simulink model "MAIN_SAT_PID"  (R2018b)
settings: Solver=FixedStepAuto  StartTime=0.0  StopTime=10.0  FixedStep=0.01  RelTol=1e-3
libraries: simulink x3
settings Model: Creator=22672  LastModifiedBy=cx

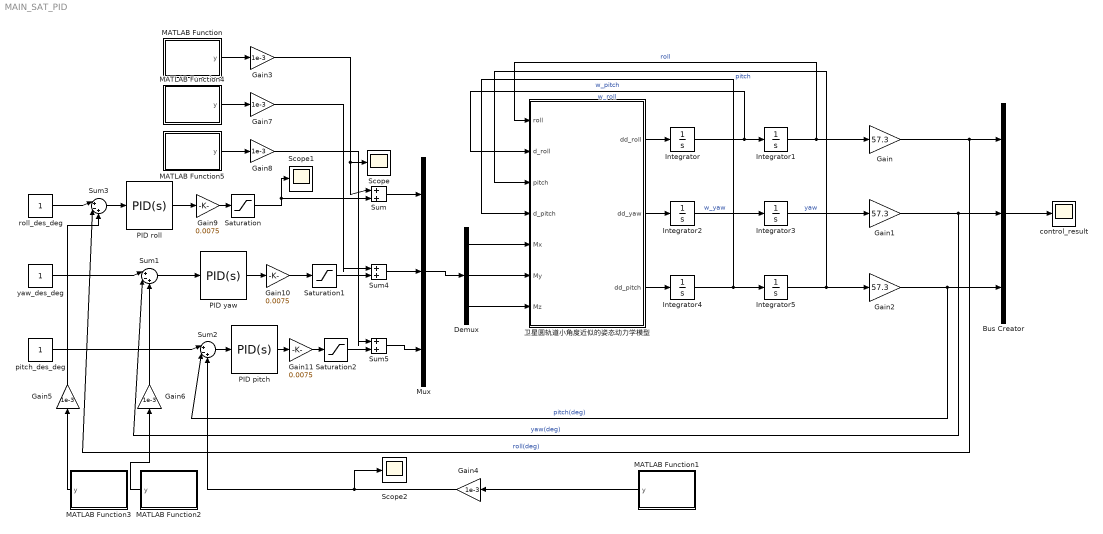
== system MAIN_SAT_PID ==
  Bus Creator : BusCreator  Inputs=3
  Demux : Demux  Outputs=3
  Gain : Gain  Gain=57.3
  Gain1 : Gain  Gain=57.3
  Gain10 : Gain  Gain=0.0075
  Gain11 : Gain  Gain=0.0075
  Gain2 : Gain  Gain=57.3
  Gain{3..8} (6 alike) : Gain  Gain=1e-3
  Gain9 : Gain  Gain=0.0075
  Integrator{,1..5} (6 alike) : Integrator
  MATLAB Function : MATLAB Function  TreatAsAtomicUnit=on
  MATLAB Function1 : MATLAB Function  TreatAsAtomicUnit=on
  MATLAB Function2 : MATLAB Function  TreatAsAtomicUnit=on
  MATLAB Function3 : MATLAB Function  TreatAsAtomicUnit=on
  MATLAB Function4 : MATLAB Function  TreatAsAtomicUnit=on
  MATLAB Function5 : MATLAB Function  TreatAsAtomicUnit=on
  Mux : Mux  Inputs=3
  PID pitch : simulink/Continuous/PID Controller  Controller=PID  Form=Parallel  TimeDomain=Continuous-time  SampleTime=-1  IntegratorMethod=Forward Euler  FilterMethod=Forward Euler  ControllerParametersSource=internal  P=22  I=0  D=14.2  UseFilter=on  N=100  TunerSelectOption=Transfer Function Based (PID Tuner App)  InitialConditionSource=internal  InitialConditionForIntegrator=0  InitialConditionForFilter=0  DifferentiatorICPrevScaledInput=0  ExternalReset=none  TrackingMode=off  Kt=1  LimitOutput=off  UpperSaturationLimit=inf  LowerSaturationLimit=-inf  LinearizeAsGain=on  AntiWindupMode=none  Kb=1  POutMin=[]  POutMax=[]  IOutMin=[]  IOutMax=[]  DOutMin=[]  DOutMax=[]  NOutMin=[]  NOutMax=[]  SumOutMin=[]  SumOutMax=[]  SaturationOutMin=[]  SaturationOutMax=[]  PParamMin=[]  PParamMax=[]  IParamMin=[]  IParamMax=[]  DParamMin=[]  DParamMax=[]  NParamMin=[]  NParamMax=[]  KbParamMin=[]  KbParamMax=[]  KtParamMin=[]  KtParamMax=[]  KbOutMin=[]  KbOutMax=[]  KtOutMin=[]  KtOutMax=[]  IntegratorOutMin=[]  IntegratorOutMax=[]  FilterOutMin=[]  FilterOutMax=[]  SumI1OutMin=[]  SumI1OutMax=[]  SumI2OutMin=[]  SumI2OutMax=[]  SumI3OutMin=[]  SumI3OutMax=[]  SumI4OutMin=[]  SumI4OutMax=[]  SumDOutMin=[]  SumDOutMax=[]  DifferentiatorOutMin=[]  DifferentiatorOutMax=[]  FilterDiffOutCoefMin=[]  FilterDiffOutCoefMax=[]  ReciprocalOutMin=[]  ReciprocalOutMax=[]  SumDenOutMin=[]  SumDenOutMax=[]  SumNumOutMin=[]  SumNumOutMax=[]  DivideOutMin=[]  DivideOutMax=[]  IntegratorContinuousStateAttributes=''  IntegratorStateMustResolveToSignalObject=off  IntegratorRTWStateStorageClass=Auto  FilterContinuousStateAttributes=''  FilterStateMustResolveToSignalObject=off  FilterRTWStateStorageClass=Auto  ParallelPVariant=InternalParameters  IdealPVariant=Disabled  IVariant=InternalParameters  DVariant=InternalParameters  IntegratorVariant=Continuous  SatVariant=Disabled  AWVariant=Passthrough  PCopyVariant=Disabled  TRVariant=Disabled  FdbkBlocksVariant=Forward  IdealPFdbkVariant=Disabled  SatFdbkVariant=Disabled  DerivativeFilterVariant=ContFilter  NVariant=InternalParameters  NCopyVariant=Disabled  FilterICVariant=InternalICsFilter  IntegratorICVariant=InternalICs  ExternalResetVariant=Disabled  TRSumVariant=Passthrough  SumFdbkVariant=Disabled  SumVariant=Sum_PID
  PID roll : simulink/Continuous/PID Controller  Controller=PID  Form=Parallel  TimeDomain=Continuous-time  SampleTime=-1  IntegratorMethod=Forward Euler  FilterMethod=Forward Euler  ControllerParametersSource=internal  P=40  I=0  D=12  UseFilter=on  N=100  TunerSelectOption=Transfer Function Based (PID Tuner App)  InitialConditionSource=internal  InitialConditionForIntegrator=0  InitialConditionForFilter=0  DifferentiatorICPrevScaledInput=0  ExternalReset=none  TrackingMode=off  Kt=1  LimitOutput=off  UpperSaturationLimit=inf  LowerSaturationLimit=-inf  LinearizeAsGain=on  AntiWindupMode=none  Kb=1  POutMin=[]  POutMax=[]  IOutMin=[]  IOutMax=[]  DOutMin=[]  DOutMax=[]  NOutMin=[]  NOutMax=[]  SumOutMin=[]  SumOutMax=[]  SaturationOutMin=[]  SaturationOutMax=[]  PParamMin=[]  PParamMax=[]  IParamMin=[]  IParamMax=[]  DParamMin=[]  DParamMax=[]  NParamMin=[]  NParamMax=[]  KbParamMin=[]  KbParamMax=[]  KtParamMin=[]  KtParamMax=[]  KbOutMin=[]  KbOutMax=[]  KtOutMin=[]  KtOutMax=[]  IntegratorOutMin=[]  IntegratorOutMax=[]  FilterOutMin=[]  FilterOutMax=[]  SumI1OutMin=[]  SumI1OutMax=[]  SumI2OutMin=[]  SumI2OutMax=[]  SumI3OutMin=[]  SumI3OutMax=[]  SumI4OutMin=[]  SumI4OutMax=[]  SumDOutMin=[]  SumDOutMax=[]  DifferentiatorOutMin=[]  DifferentiatorOutMax=[]  FilterDiffOutCoefMin=[]  FilterDiffOutCoefMax=[]  ReciprocalOutMin=[]  ReciprocalOutMax=[]  SumDenOutMin=[]  SumDenOutMax=[]  SumNumOutMin=[]  SumNumOutMax=[]  DivideOutMin=[]  DivideOutMax=[]  IntegratorContinuousStateAttributes=''  IntegratorStateMustResolveToSignalObject=off  IntegratorRTWStateStorageClass=Auto  FilterContinuousStateAttributes=''  FilterStateMustResolveToSignalObject=off  FilterRTWStateStorageClass=Auto  ParallelPVariant=InternalParameters  IdealPVariant=Disabled  IVariant=InternalParameters  DVariant=InternalParameters  IntegratorVariant=Continuous  SatVariant=Disabled  AWVariant=Passthrough  PCopyVariant=Disabled  TRVariant=Disabled  FdbkBlocksVariant=Forward  IdealPFdbkVariant=Disabled  SatFdbkVariant=Disabled  DerivativeFilterVariant=ContFilter  NVariant=InternalParameters  NCopyVariant=Disabled  FilterICVariant=InternalICsFilter  IntegratorICVariant=InternalICs  ExternalResetVariant=Disabled  TRSumVariant=Passthrough  SumFdbkVariant=Disabled  SumVariant=Sum_PID
  PID yaw : simulink/Continuous/PID Controller  Controller=PID  Form=Parallel  TimeDomain=Continuous-time  SampleTime=-1  IntegratorMethod=Forward Euler  FilterMethod=Forward Euler  ControllerParametersSource=internal  P=30  I=0  D=13.67  UseFilter=on  N=100  TunerSelectOption=Transfer Function Based (PID Tuner App)  InitialConditionSource=internal  InitialConditionForIntegrator=0  InitialConditionForFilter=0  DifferentiatorICPrevScaledInput=0  ExternalReset=none  TrackingMode=off  Kt=1  LimitOutput=off  UpperSaturationLimit=inf  LowerSaturationLimit=-inf  LinearizeAsGain=on  AntiWindupMode=none  Kb=1  POutMin=[]  POutMax=[]  IOutMin=[]  IOutMax=[]  DOutMin=[]  DOutMax=[]  NOutMin=[]  NOutMax=[]  SumOutMin=[]  SumOutMax=[]  SaturationOutMin=[]  SaturationOutMax=[]  PParamMin=[]  PParamMax=[]  IParamMin=[]  IParamMax=[]  DParamMin=[]  DParamMax=[]  NParamMin=[]  NParamMax=[]  KbParamMin=[]  KbParamMax=[]  KtParamMin=[]  KtParamMax=[]  KbOutMin=[]  KbOutMax=[]  KtOutMin=[]  KtOutMax=[]  IntegratorOutMin=[]  IntegratorOutMax=[]  FilterOutMin=[]  FilterOutMax=[]  SumI1OutMin=[]  SumI1OutMax=[]  SumI2OutMin=[]  SumI2OutMax=[]  SumI3OutMin=[]  SumI3OutMax=[]  SumI4OutMin=[]  SumI4OutMax=[]  SumDOutMin=[]  SumDOutMax=[]  DifferentiatorOutMin=[]  DifferentiatorOutMax=[]  FilterDiffOutCoefMin=[]  FilterDiffOutCoefMax=[]  ReciprocalOutMin=[]  ReciprocalOutMax=[]  SumDenOutMin=[]  SumDenOutMax=[]  SumNumOutMin=[]  SumNumOutMax=[]  DivideOutMin=[]  DivideOutMax=[]  IntegratorContinuousStateAttributes=''  IntegratorStateMustResolveToSignalObject=off  IntegratorRTWStateStorageClass=Auto  FilterContinuousStateAttributes=''  FilterStateMustResolveToSignalObject=off  FilterRTWStateStorageClass=Auto  ParallelPVariant=InternalParameters  IdealPVariant=Disabled  IVariant=InternalParameters  DVariant=InternalParameters  IntegratorVariant=Continuous  SatVariant=Disabled  AWVariant=Passthrough  PCopyVariant=Disabled  TRVariant=Disabled  FdbkBlocksVariant=Forward  IdealPFdbkVariant=Disabled  SatFdbkVariant=Disabled  DerivativeFilterVariant=ContFilter  NVariant=InternalParameters  NCopyVariant=Disabled  FilterICVariant=InternalICsFilter  IntegratorICVariant=InternalICs  ExternalResetVariant=Disabled  TRSumVariant=Passthrough  SumFdbkVariant=Disabled  SumVariant=Sum_PID
  Saturation : Saturate  UpperLimit=0.1  LowerLimit=-0.1
  Saturation1 : Saturate  UpperLimit=0.1  LowerLimit=-0.1
  Saturation2 : Saturate  UpperLimit=0.1  LowerLimit=-0.1
  Scope : Scope
  Scope1 : Scope
  Scope2 : Scope
  Sum : Sum  Inputs=|++
  Sum1 : Sum  Inputs=|+-+
  Sum2 : Sum  Inputs=|+-+
  Sum3 : Sum  Inputs=|+-+
  Sum4 : Sum  Inputs=|++
  Sum5 : Sum  Inputs=|++
  control_result : Scope
  pitch_des_deg : Constant
  roll_des_deg : Constant
  yaw_des_deg : Constant
  卫星圆轨道小角度近似的姿态动力学模型 : MATLAB Function  TreatAsAtomicUnit=on
  wires:
  Integrator2/1 -> Integrator3/1  "w_yaw"
  Gain2/1 -> Bus Creator/3, Sum2/2  "pitch(deg)"
  Integrator3/1 -> Gain1/1  "yaw"
  Gain/1 -> Sum3/2, Bus Creator/1  "roll(deg)"
  Integrator4/1 -> Integrator5/1, 卫星圆轨道小角度近似的姿态动力学模型/4(d_pitch)  "w_pitch"
  Integrator/1 -> Integrator1/1, 卫星圆轨道小角度近似的姿态动力学模型/2(d_roll)  "w_roll"
  Gain1/1 -> Bus Creator/2, Sum1/2  "yaw(deg)"
  卫星圆轨道小角度近似的姿态动力学模型/2(dd_yaw) -> Integrator2/1
  Bus Creator/1 -> control_result/1
  卫星圆轨道小角度近似的姿态动力学模型/3(dd_pitch) -> Integrator4/1
  Integrator5/1 -> 卫星圆轨道小角度近似的姿态动力学模型/3(pitch), Gain2/1  "pitch"
  Integrator1/1 -> 卫星圆轨道小角度近似的姿态动力学模型/1(roll), Gain/1  "roll"
  卫星圆轨道小角度近似的姿态动力学模型/1(dd_roll) -> Integrator/1
  Demux/3 -> 卫星圆轨道小角度近似的姿态动力学模型/7(Mz)
  Demux/2 -> 卫星圆轨道小角度近似的姿态动力学模型/6(My)
  Demux/1 -> 卫星圆轨道小角度近似的姿态动力学模型/5(Mx)
  Mux/1 -> Demux/1
  Sum/1 -> Mux/1
  MATLAB Function/1(y) -> Gain3/1
  Sum1/1 -> PID yaw/1
  Sum2/1 -> PID pitch/1
  yaw_des_deg/1 -> Sum1/1
  Sum3/1 -> PID roll/1
  roll_des_deg/1 -> Sum3/1
  pitch_des_deg/1 -> Sum2/1
  Gain3/1 -> Scope/1, Sum/1
  Saturation/1 -> Scope1/1, Sum/2
  MATLAB Function1/1(y) -> Gain4/1
  Gain4/1 -> Scope2/1, Sum2/3
  MATLAB Function2/1(y) -> Gain6/1
  MATLAB Function3/1(y) -> Gain5/1
  Gain5/1 -> Sum3/3
  Gain6/1 -> Sum1/3
  Sum4/1 -> Mux/2
  Saturation1/1 -> Sum4/2
  Sum5/1 -> Mux/3
  Saturation2/1 -> Sum5/2
  Gain7/1 -> Sum4/1
  MATLAB Function4/1(y) -> Gain7/1
  MATLAB Function5/1(y) -> Gain8/1
  Gain8/1 -> Sum5/1
  PID roll/1 -> Gain9/1
  Gain9/1 -> Saturation/1
  PID yaw/1 -> Gain10/1
  Gain10/1 -> Saturation1/1
  PID pitch/1 -> Gain11/1
  Gain11/1 -> Saturation2/1

== matlab function MAIN_SAT_PID/MATLAB Function ==
  data: y output
function y = disturb()
y=wgn(1,1,1);

== matlab function MAIN_SAT_PID/卫星圆轨道小角度近似的姿态动力学模型 ==
  data: roll input; d_roll input; pitch input; d_pitch input; dd_roll output; dd_yaw output; dd_pitch output; Mx input; My input; Mz input
function [dd_roll,dd_yaw,dd_pitch] = satelite(roll,d_roll,pitch,d_pitch,Mx,My,Mz)
%航天器小角度近似姿态动力学模型 圆轨道假设、小角度假设
%Y = [滚转角速度，偏航角速度，俯仰角速度，滚转角，偏航角，俯仰角]，Cx(滚转) Cz(俯仰) Cy(偏航)
%主轴转动惯量
Ix = 0.533;
Iy = 0.533*2;
Iz = 0.533*3;
mu_e = 3.986e14;%地球引力常数m^3/s^-2
H = 500e3;%卫星轨道高度m
R = 6378e3;%地球赤道平均半径m

%动力学模型
w0 = sqrt(mu_e/(R+H)^3);%圆轨道角速度
dd_roll = ( Mx - (Iy-Iz-Ix) * w0 * d_pitch - (Iy-Iz) * w0 * w0 * roll) / Ix;
dd_yaw = My / Iy;
dd_pitch = ( Mz + (Iy-Iz-Ix) * w0 * d_roll - (Iy-Ix) * w0 * w0 * pitch ) / Iz;

== matlab function MAIN_SAT_PID/MATLAB Function1 ==
  data: y output
function y = noise()
y=wgn(1,1,1);

== matlab function MAIN_SAT_PID/MATLAB Function2 ==
  data: y output
function y = noise()
y=wgn(1,1,1);

== matlab function MAIN_SAT_PID/MATLAB Function3 ==
  data: y output
function y = noise()
y=wgn(1,1,1);

== matlab function MAIN_SAT_PID/MATLAB Function4 ==
  data: y output
function y = disturb()
y=wgn(1,1,1);

== matlab function MAIN_SAT_PID/MATLAB Function5 ==
  data: y output
function y = disturb()
y=wgn(1,1,1);
